simulink model "sf_tlat"  (Simulink 6.0)
settings: Solver=ode45  StartTime=0.0  StopTime=100  RelTol=1e-3
settings Model: CovMetricSettings=dcmtr  Creator=The MathWorks Inc.  LastModifiedBy=batserve  ExtModeAutoUpdateStatusClock=off
settings OptimizationCC: BooleanDataType=off
settings DebuggingCC: CheckExecutionContextPreStartOutputMsg=on  CheckExecutionContextRuntimeOutputMsg=on  SolverPrmCheckMsg=none
settings HardwareCC: TargetUnknown=on

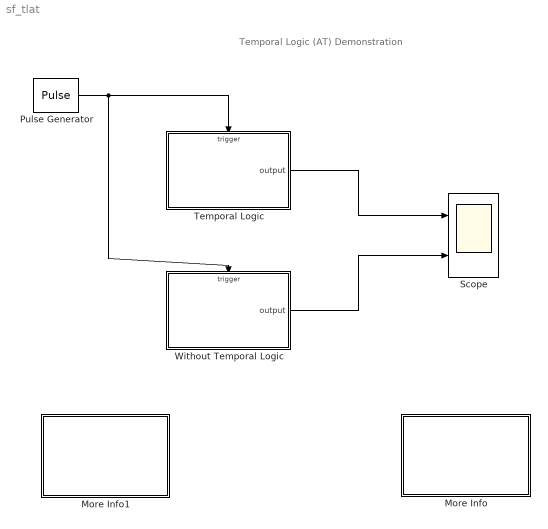
== system sf_tlat ==
  note: Temporal Logic (AT) Demonstration
  More Info : Subsystem  PropExecContextAcrossSSBoundary=on
      mask Display: disp('Double click\nhere for\ninformation on\nthis demonstration')
  More Info1 : Subsystem  PropExecContextAcrossSSBoundary=on
      settings: OpenFcn=simcad(bdroot);
      mask Display: disp('Double click\nhere for\nSimulink\Stateflow\n Help')
  Pulse Generator : DiscretePulseGenerator  PulseType=Time based  Period=1  PulseWidth=50
  Scope : Scope  NumInputPorts=2
      settings: TimeRange=100  YMin=-1.5~-1.5  YMax=1.5~1.5
  Temporal Logic : Stateflow chart  TreatAsAtomicUnit=on  PropExecContextAcrossSSBoundary=on
  Without Temporal Logic : Stateflow chart  TreatAsAtomicUnit=on  PropExecContextAcrossSSBoundary=on
  wires:
  Pulse Generator/1 -> Temporal Logic/Trigger, Without Temporal Logic/Trigger
  Temporal Logic/1(output) -> Scope/1
  Without Temporal Logic/1(output) -> Scope/2

== system sf_tlat/More Info ==
  note: Temporal Logic using the AT function
  note: In this demo, we illustrate the advantage of using the AT function. In this demo, the AT function is
      | used three times in the 'Temporal Logic' chart. After setting a value a=5, we use the AT function to
      | change the final output in the chart. On the 5th ('a') event, we set the output to 1; on the 10th ('2*a')
      | event, we set the output to 0; and finally, on the 30th ('6*a') event we set the output to equal -1.
      |
      | In the 'Without Temporal Logic' chart, we need to use many more states and transitions to create
      | the same model. We also needed to create an extra local variable, 'count', to be used as a counter
      | for every occurrence. In general, there were many more definitions and declarations needed to
      | create the same model without using temporal logic. This increases the chance for error as well
      | as the size of the generated code.

== system sf_tlat/More Info1 ==

== stateflow chart Temporal Logic ==
  state State
    a=5;
    on at(a,event):output=1;
    on at(2*a,event):output=0;
  (default) -> State
  State -> (junction 4) : at(6*a,event)
  (junction 4) -> State : {output=-1;}
  data: output output double; a local double
  events: event input RISING_EDGE_EVENT

== stateflow chart Without Temporal Logic ==
  state A
    en: count = 1;
    A -> A : {count++;a=count;}
  state B
    en:count=a+1;
    B -> B : {count++;}
  state C
    en:count=2*a+1;
    C -> C : {count++;}
  (default) -> A
  A -> B : [count==5]{output=1;}
  B -> C : [count==2*a]{output=0;}
  C -> A : [count==6*a]{output=-1;}
  data: count local double; output output double; a local double
  events: control input RISING_EDGE_EVENT
